simulink model "Tema_bonus_Pisai_Daria_PC5_2"  (R2024b)
settings: Solver=FixedStepAuto  StartTime=0.0  StopTime=1000  FixedStep=0.01  RelTol=1e-3
settings Model: Creator=dariapisai  LastModifiedBy=dariapisai

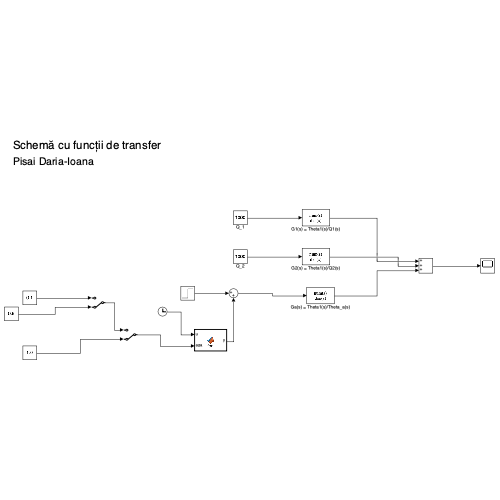
[thumbnail: Simulink's stored preview of the top-level diagram]
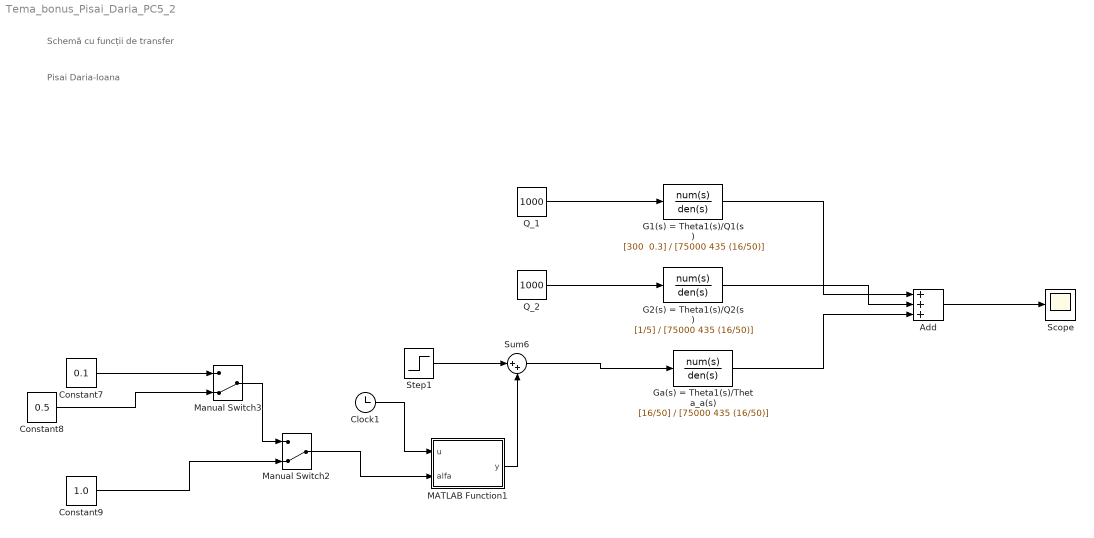
== system Tema_bonus_Pisai_Daria_PC5_2 ==
  note: Pisai Daria-Ioana
  note: Schemă cu funcții de transfer
  Add : Sum  Inputs=+++
  Clock1 : Clock
      settings: Decimation=1000
  Constant7 : Constant  Value=0.1
  Constant8 : Constant  Value=0.5
  Constant9 : Constant  Value=1.0
  G1(s) = Theta1(s)/Q1(s) : TransferFcn  Numerator="[300  0.3]"  Denominator=[75000 435 (16/50)]
  G2(s) = Theta1(s)/Q2(s) : TransferFcn  Numerator=[1/5]  Denominator=[75000 435 (16/50)]
  Ga(s) = Theta1(s)/Theta_a(s) : TransferFcn  Numerator=[16/50]  Denominator=[75000 435 (16/50)]
  MATLAB Function1 : MATLAB Function  TreatAsAtomicUnit=on
  Manual Switch2 : ManualSwitch  CurrentSetting=0
  Manual Switch3 : ManualSwitch  CurrentSetting=0
  Q_1 : Constant  Value=1000
  Q_2 : Constant  Value=1000
  Scope : Scope
  Step1 : Step  Time=5  SampleTime=0
  Sum6 : Sum  Inputs=|++
  wires:
  Step1/1 -> Sum6/1
  Manual Switch3/1 -> Manual Switch2/1
  Sum6/1 -> Ga(s) = Theta1(s)/Theta_a(s)/1
  Ga(s) = Theta1(s)/Theta_a(s)/1 -> Add/3
  Clock1/1 -> MATLAB Function1/1(u)
  Constant9/1 -> Manual Switch2/2
  G2(s) = Theta1(s)/Q2(s)/1 -> Add/2
  MATLAB Function1/1(y) -> Sum6/2
  Add/1 -> Scope/1
  Constant8/1 -> Manual Switch3/2
  Manual Switch2/1 -> MATLAB Function1/2(alfa)
  Constant7/1 -> Manual Switch3/1
  Q_2/1 -> G2(s) = Theta1(s)/Q2(s)/1
  G1(s) = Theta1(s)/Q1(s)/1 -> Add/1
  Q_1/1 -> G1(s) = Theta1(s)/Q1(s)/1

== matlab function Tema_bonus_Pisai_Daria_PC5_2/MATLAB Function1 ==
  data: u input; y output; alfa input
function y = fcn(u, alfa)

A = 2;

y = A*exp((-alfa)*u);

end
